simulink model "feedback_plant"  (R2020b)
settings: Solver=ode45  StartTime=0.0  StopTime=10.0  MaxStep=0.1  RelTol=1e-3  EnableMultiTasking=on
settings Model: ModifiedByFormat=The MathWorks Inc.  Creator=The MathWorks, Inc.  LastModifiedBy=The MathWorks Inc.
settings DataIOCC: SaveFormat=Array  ReturnWorkspaceOutputs=off
settings OptimizationCC: DefaultParameterBehavior=Inlined  ExpressionDepthLimit=2147483647  LifeSpan=1
settings DebuggingCC: UnderspecifiedInitializationDetection=Classic  MergeDetectMultiDrivingBlocksExec=none  SolverPrmCheckMsg=warning  FcnCallInpInsideContextMsg=warning  AllowSymbolicDim=off  StateNameClashWarn=warning  SFUnexpectedBacktrackingDiag=warning  SFNoUnconditionalDefaultTransitionDiag=warning  SFExecutionAtInitializationDiag=none  ArithmeticOperatorsInVariantConditions=warning
settings HardwareCC: ProdBitPerPointer=32  ProdBitPerSizeT=32  ProdBitPerPtrDiffT=32  ProdLargestAtomicFloat=None  ProdIntDivRoundTo=Undefined  ProdEndianess=Unspecified  ProdWordSize=32  ProdHWDeviceType=32-bit Generic
settings ModelReferenceCC: PropagateSignalLabelsOutOfModel=off
settings SFSimCC: SimUseLocalCustomCode=off  CustomCodeUndefinedFunction=UseInterfaceOnly
settings RTWCC: RTWUseLocalCustomCode=off
settings CodeAppCC: StateflowObjectComments=on
settings GRTTargetCC: TargetLangStandard=C89/C90 (ANSI)  CombineOutputUpdateFcns=off  GRTInterface=on
settings ConfigComp: CovMetricSettings=dw  CovSaveCumulativeToWorkspaceVar=on  CovSaveSingleToWorkspaceVar=on  CovExternalEMLEnable=off  CovSFcnEnable=off

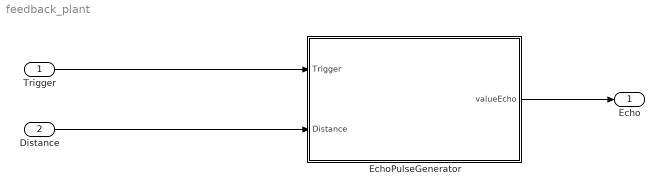
== system feedback_plant ==
  Trigger : Inport  OutDataTypeStr=boolean
  Distance : Inport  Port=2  OutDataTypeStr=double
  EchoPulseGenerator : Stateflow chart  TreatAsAtomicUnit=on
  Echo : Outport  OutDataTypeStr=double
  wires:
  Distance/1 -> EchoPulseGenerator/2(Distance)
  EchoPulseGenerator/1(valueEcho) -> Echo/1
  Trigger/1 -> EchoPulseGenerator/1(Trigger)

== stateflow chart feedback_plant/EchoPulseGenerator ==
  state WAIT_TO_RISE
  state WAIT_TO_FALL
  note: If no measurement is detected, the Echo signal is not generated
  note: Wait trigger low before generating the Echo
  state WAIT_TRIGGER_LOW
  state ENABLED
    state HIGH
      en: valueEcho=1;
    state LOW
      en: valueEcho=0;
    (default) -> HIGH
    HIGH -> LOW : after((Distance*58),usec)
  (default) -> WAIT_TO_RISE
  (junction 29) -> WAIT_TO_RISE
  (junction 27) -> (junction 29)
  WAIT_TO_RISE -> WAIT_TO_FALL : [Trigger==1]
  WAIT_TO_FALL -> (junction 27) [order 2] : [Trigger==0]
  (junction 34) -> (junction 27)
  WAIT_TO_FALL -> WAIT_TRIGGER_LOW [order 1] : after(10,usec)[Distance~=0]
  WAIT_TRIGGER_LOW -> ENABLED : [Trigger==0]
  ENABLED -> (junction 34) : [valueEcho==0]
  data: Trigger input boolean; Distance input double; valueEcho output double
